simulink model "psbbridges"  (Simulink 6.0)
settings: Solver=FixedStepDiscrete  StartTime=0.0  StopTime=0.10  FixedStep=Ts  RelTol=1e-3  AbsTol=1e-3
PreLoadFcn:
  | assignin('base','Ts',[2e-6])
InitFcn:
  | powericon('psbinitsys',bdroot);
undefined symbols (not defined in the file or in its folder): D1, Delta, Ts
libraries: powerlib2 x16, powerlib_extras x5
settings Model: Creator=sybille  LastModifiedBy=batserve  ExtModeTrigMode=oneshot  ExtModeArmWhenConnect=off  ExtModeAutoUpdateStatusClock=off
settings DataIOCC: LimitDataPoints=off  SaveOutput=off  SaveTime=off  SignalLoggingName=sigsOut
settings OptimizationCC: BlockReduction=off  BooleanDataType=off
settings DebuggingCC: CheckExecutionContextPreStartOutputMsg=on  CheckExecutionContextRuntimeOutputMsg=on  SolverPrmCheckMsg=none
settings HardwareCC: TargetUnknown=on

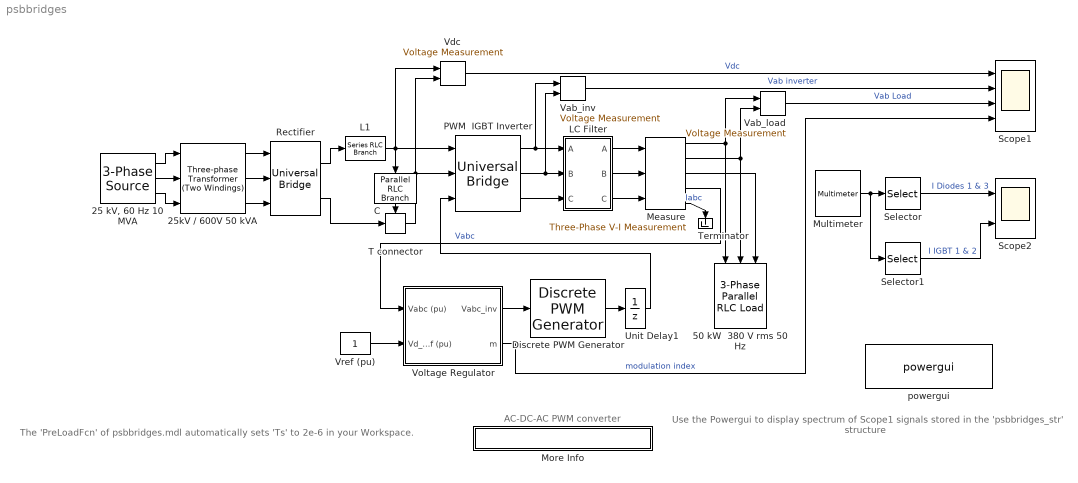
== system psbbridges ==
  note: AC-DC-AC PWM converter
  note: The 'PreLoadFcn' of psbbridges.mdl
      | automatically sets 'Ts' to 2e-6 in your Workspace.
  note: Use the Powergui to display
      | spectrum of Scope1 signals
      | stored in the  'psbbridges_str'
      | structure
  "25 kV, 60 Hz 10 MVA" : powerlib2/Electrical Sources/3-Phase Source  Tag=PoWeRsYsTeMbLoCk  V=25e3  Phi=0  F=60  InternalConnection=Yg  RLoff=on  R=25e3^2/10e6/5  L=25e3^2/10e6/377  Psc=10e6  Vbase=25e3  XRratio=5  PSBOutputType=111
  25kV / 600V 50 kVA : powerlib2/Elements/Three-phase Transformer (Two Windings)  Tag=PoWeRsYsTeMbLoCk  nominal=[ 50e3 , 60 ]  type1=Yg  params1=[ 25e3 , 0.004 , 0.02 ]  type2=Delta (D1)  params2=[ 600 , 0.004 , 0.02 ]  ynsat=off  rmag=200  lm=200  sat="[ 0,0  ;  0.005,1.2  ;  1.0,1.4 ]"  hyst=off  matfile='hysteresis'  sif=off  phi0=[ 0.8 , -0.8 , 0.7 ]  initialslopes=[+1 +1 +1]  mesure=None  PSBOutputType=1111
  50 kW  380 V rms 50 Hz : powerlib2/Elements/3-Phase Parallel RLC Load  Orientation=down  Vpp=380  fn=50  P3=50e3  QL3=0  QC3=0
  C : powerlib2/Elements/Parallel RLC Branch  Tag=PoWeRsYsTeMbLoCk  Orientation=down  a=inf  b=inf  c=5000e-06  mesure=None  PSBOutputType=1
  Discrete PWM Generator : powerlib_extras/Discrete  Control Blocks/Discrete PWM Generator  GeneratorMode="3-arm  bridge (6 pulses)"  Fc=2000  Ts=Ts  Internal=off  mIndex=0.4  Freq=60  Phase=0
  L1 : powerlib2/Elements/Series RLC Branch  Tag=PoWeRsYsTeMbLoCk  a=0  b=200e-6  c=inf  mesure=None  PSBOutputType=1
  LC Filter : Subsystem
  Measure : powerlib2/Measurements/Three-Phase V-I Measurement  Tag=PoWeRsYsTeMmEaSuReMeNt  VChoice=phase-to-ground  ualv=off  labelV=V1  Vpu=on  Vbase=380  IChoice=yes  ualc=off  labelC=I1  Ppu=off  Pbase=1e3  OutputType=Magnitude  PhasorSimulation=off  PSBequivalent=0  PSBOutputType=11100
  More Info : Subsystem
      mask Display: disp('? : Double click here for more info')
  Multimeter : powerlib2/Measurements/Multimeter  Tag=PoWeRsYsTeMmEaSuReMeNt  PhasorSimulation=off  OutputType=Magnitude  sel=[1 3 7 8]  L=12  Gain=[1 1 1 1]  yselected="{'Isw1: Rectifier','Isw3: Rectifier','Isw1: PWM  IGBT Inverter','Isw2: PWM  IGBT Inverter'};"  PSBOutputType=1  PSBequivalent=0  AxesSetting=[0,0.1,-100,100]  Display=0  SavedBlockNames=-11
  PWM  IGBT Inverter : powerlib2/Power Electronics/Universal Bridge  Tag=PoWeRsYsTeMbLoCk  arms=3  confi=ABC as output terminals  injcc=5000  cf=inf  device=IGBT / Diodes  Ron=1e-3  Lon=0  VFs="[  0.0  0.0  ]"  Vf=.8  gtoparameters=[ 1e-6 ,1e-6 ]  igbtparameters=[ 1e-6 , 2e-6 ]  mesure=Device currents  PSBOutputType=111
  Rectifier : powerlib2/Power Electronics/Universal Bridge  Tag=PoWeRsYsTeMbLoCk  arms=3  confi=ABC as input terminals  injcc=100  cf=0.1e-6  device=Diodes  Ron=1e-3  Lon=0  VFs="[  0.8  0.8  ]"  Vf=.8  gtoparameters=[ 10e-6 , 20e-6 ]  igbtparameters=[ 1e-6 , 2e-6 ]  mesure=Device currents  PSBOutputType=111
  Scope1 : Scope  NumInputPorts=4
      settings: TimeRange=0.1  YMin=0~-1500~-750~0.4  YMax=1100~1500~750~1.1  SaveName=psbbridges_str
  Scope2 : Scope  NumInputPorts=2
      settings: TimeRange=0.09999999999999999  YMin=-10~-125  YMax=100~125
  Selector : Selector  Elements=[1 2]  InputPortWidth=4
  Selector1 : Selector  Elements=[3 4]  InputPortWidth=4
  T connector : powerlib2/Connectors/T connector  Tag=PoWeRsYsTeMbLoCk  PSBOutputType=1
  Terminator : Terminator
      settings: Orientation=down
  Unit Delay1 : UnitDelay  SampleTime=Ts
  Vab_inv : powerlib2/Measurements/Voltage Measurement  Tag=PoWeRsYsTeMmEaSuReMeNt  PhasorSimulation=off  OutputType=Magnitude  PSBOutputType=0  PSBequivalent=0
  Vab_load : powerlib2/Measurements/Voltage Measurement  Tag=PoWeRsYsTeMmEaSuReMeNt  PhasorSimulation=off  OutputType=Magnitude  PSBOutputType=0  PSBequivalent=0
  Vdc : powerlib2/Measurements/Voltage Measurement  Tag=PoWeRsYsTeMmEaSuReMeNt  PhasorSimulation=off  OutputType=Magnitude  PSBOutputType=0  PSBequivalent=0
  Voltage Regulator : Subsystem  mask( Voltage Regulator){Kp=0.4, Ki=500, Ts=Ts}
      mask prompts: Kp "Proportional gain  Kp:"; Ki "Integral gain Ki:"; Ts "Sample time (s) :"
  "Vref (pu) " : Constant
  powergui : powerlib2/powergui  Frange=[0:2:500]  Ylog=off  Xlog=on  save=off  variable=ZData  structure=psbbridges_str  ZoomFFT=on  StartTime=0.1-2/50  cycles=2  DisplayStyle=off  fundamental=50  FreqAxis=off  MaxFrequency=7000  frequencyindice=1  frequencyindicesteady=1  RmsSteady=1  display=off  Ts=Ts  methode=off  frequency=60  echomessages=off
  wires:
  C/1 -> T connector/Enable
  T connector/1 -> PWM  IGBT Inverter/2, Vdc/2
  L1/1 -> PWM  IGBT Inverter/1, C/1, Vdc/1
  25kV / 600V 50 kVA/3 -> Rectifier/3
  "25 kV, 60 Hz 10 MVA"/1 -> 25kV / 600V 50 kVA/1
  "25 kV, 60 Hz 10 MVA"/2 -> 25kV / 600V 50 kVA/2
  "25 kV, 60 Hz 10 MVA"/3 -> 25kV / 600V 50 kVA/3
  25kV / 600V 50 kVA/2 -> Rectifier/2
  PWM  IGBT Inverter/1 -> Vab_inv/1, LC Filter/1(A)
  PWM  IGBT Inverter/2 -> Vab_inv/2, LC Filter/2(B)
  PWM  IGBT Inverter/3 -> LC Filter/3(C)
  LC Filter/1("A ") -> Measure/1
  LC Filter/2("B ") -> Measure/2
  LC Filter/3("C ") -> Measure/3
  Measure/3 -> 50 kW  380 V rms 50 Hz/3
  Measure/1 -> 50 kW  380 V rms 50 Hz/1, Vab_load/1
  Measure/2 -> 50 kW  380 V rms 50 Hz/2, Vab_load/2
  Measure/4 -> Voltage Regulator/1(Vabc (pu))  "Vabc"
  "Vref (pu) "/1 -> Voltage Regulator/2(Vd_ref (pu))
  Selector/1 -> Scope2/1  "I Diodes 1 & 3"
  Multimeter/1 -> Selector/1, Selector1/1
  Selector1/1 -> Scope2/2  "I IGBT 1 & 2"
  Measure/5 -> Terminator/1  "Iabc"
  25kV / 600V 50 kVA/1 -> Rectifier/1
  Rectifier/1 -> L1/1
  Rectifier/2 -> T connector/1
  Discrete PWM Generator/1 -> Unit Delay1/1
  Unit Delay1/1 -> PWM  IGBT Inverter/3
  Voltage Regulator/1(Vabc_inv) -> Discrete PWM Generator/1
  Voltage Regulator/2(m) -> Scope1/4  "modulation index"
  Vdc/1 -> Scope1/1  "Vdc"
  Vab_load/1 -> Scope1/3  "Vab Load"
  Vab_inv/1 -> Scope1/2  "Vab inverter"

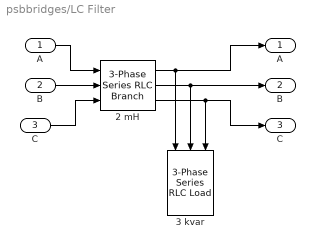
== system psbbridges/LC Filter ==
  A : Inport  Port=1  LatchInput=off
  B : Inport  Port=2  LatchInput=off
  C : Inport  Port=3  LatchInput=off
  "2 mH " : powerlib2/Elements/3-Phase Series RLC Branch   R=0  L=2e-3  C=inf
  3 kvar : powerlib2/Elements/3-Phase Series RLC Load  Orientation=down  Vpp=380  fn=50  P3=0  QL3=0  QC3=3e3
  "A " : Outport
  "B " : Outport  Port=2
  "C " : Outport  Port=3
  wires:
  B/1 -> "2 mH "/2
  A/1 -> "2 mH "/1
  C/1 -> "2 mH "/3
  "2 mH "/1 -> "A "/1, 3 kvar/1
  "2 mH "/2 -> "B "/1, 3 kvar/2
  "2 mH "/3 -> "C "/1, 3 kvar/3

== system psbbridges/More Info ==
  note: This example of AC-DC-AC converter illustrates use of Universal Bridge,
      |  Multimeter and Powergui  blocks as well as discrete control blocks of the Extras library
  note: Circuit Description
  note: Demonstration
  note: A  60 Hz, voltage source feeds a 50 Hz, 50 kW load through an  AC-DC-AC  converter.
      |
      | The 600V, 60 Hz voltage obtained at secondary of the Wye/Delta transformer is first rectified by a six pulse diode bridge.
      | The filtered DC voltage is applied to an IGBT two-level inverter generating 50 Hz.
      | The IGBT inverter uses Pulse Width Modulation (PWM) at a 2 kHz carrier frequency.
      | The circuit is discretized at a sample time of 2 us
      |
      | The load voltage is regulated  at 1 pu (380 V rms) by a PI voltage regulator using abc_to_dq and dq_to_abc transfomations.
      | The first output of the voltage regulator is a vector containing the three modulating signals used by the PMW Generator
      | to generate the 6 IGBT pulses. The second output returns the modulation index.
      |
      | The Discrete 3-Phase PWM Pulse Generator  is available in the Extras/Discrete Control Blocks library.
      | The voltage regulator has been  built from blocks of the Extras/Measurements and Extras/ Discrete Control libraries
      |
      | The Multimeter block is used to observe diode and IGBT currents.
      | In order to allow further signal processing, signals displayed on  Scope1  block  (sampled at simulation sampling rate of 2us )
      | are stored in a  variable named 'psbbridges_str' (structure with time) .
  note: Start the simulation. After a transient period of approximately  50 ms, the system reaches a steady state.
      | Observe  voltage waveforms at  DC bus, inverter output  and load on Scope1.
      | The harmonics generated by the inverter around around multiples of 2 kHz are filtered by the  LC filter.
      |
      | As expected the peak value of the load voltage is 537 V (380 Vrms).
      | In steady state the mean value of the  modulation index is m = 0.80 and the mean value of the  DC  voltage is 778 V.
      | The fundamental component of 50 Hz voltage burried in the chopped inverter voltage is therefore:
      | Vab = 778 V * 0.612 * 0.80 = 381 V rms
      |
      | Once  simulation is completed, open the Powergui and select  'FFT Analysis' to display the 0 - 7000 Hz frequency spectrum of signals saved
      | in the 'psbbridges_str' structure. The FFT will be performed on  a 2-cycle window starting at t=0.1-2/50 (last 2 cycles of recording).
      | Select input labeled 'Vab Load' . Click on Display and observe the frequency spectrum of last 2 cycles.
      | Notice harmonics around multiples of the 2 kHz carrier frequency. Maximum harmonic is 1.4 % of fundamental and THD is 2%.
      |
      | Observe diode currents on trace 1 of Scope2, showing commutation from  diode 1 to diode 3.  Also observe on trace 2 currents in
      | switches 1 and 2 of the IGBT/Diode bridge (upper and lower switches connected to phase A). These two currents are complementary.
      | A positive current indicates a current flowing in the IGBT, whereas a negative current indicates a current flowing in the antiparallel diode.
  note: G. Sybille (Hydro-Quebec)

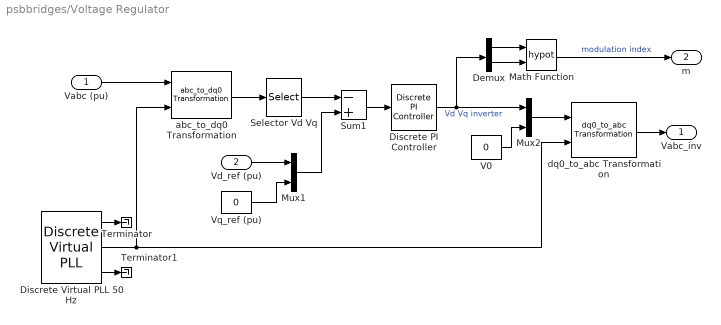
== system psbbridges/Voltage Regulator ==
  Vabc (pu) : Inport  Port=1  LatchInput=off
  Vd_ref (pu) : Inport  Port=2  LatchInput=off
  Demux : Demux  Outputs=2
  Discrete PI Controller : powerlib_extras/Discrete  Control Blocks/Discrete PI Controller  Kp=Kp  Ki=Ki  Par_Limits=[1 -1]  Init=0  Ts=Ts
  Discrete Virtual PLL 50 Hz : powerlib_extras/Discrete  Control Blocks/Discrete Virtual PLL  Freq=50  Phase=0  Ts=Ts
  Math Function : Math  Operator=hypot  SaturateOnIntegerOverflow=on
  Mux1 : Mux  Inputs=2
  Mux2 : Mux  Inputs=2
  Selector Vd Vq : Selector  Elements=[1 2]  InputPortWidth=3
  Sum1 : Sum  Inputs=-+  SaturateOnIntegerOverflow=on  InputSameDT=on
  Terminator : Terminator
  Terminator1 : Terminator
  V0 : Constant  Value=0
  Vq_ref (pu) : Constant  Value=0
  abc_to_dq0 Transformation : powerlib_extras/Measurements/abc_to_dq0 Transformation
  dq0_to_abc Transformation : powerlib_extras/Measurements/dq0_to_abc Transformation
  Vabc_inv : Outport
  m : Outport  Port=2
  wires:
  abc_to_dq0 Transformation/1 -> Selector Vd Vq/1
  Vabc (pu)/1 -> abc_to_dq0 Transformation/1
  Selector Vd Vq/1 -> Sum1/1
  Sum1/1 -> Discrete PI Controller/1
  Mux2/1 -> dq0_to_abc Transformation/1
  V0/1 -> Mux2/2
  dq0_to_abc Transformation/1 -> Vabc_inv/1
  Discrete Virtual PLL 50 Hz/2 -> abc_to_dq0 Transformation/2, dq0_to_abc Transformation/2
  Vd_ref (pu)/1 -> Mux1/1
  Vq_ref (pu)/1 -> Mux1/2
  Mux1/1 -> Sum1/2
  Discrete Virtual PLL 50 Hz/1 -> Terminator/1
  Discrete Virtual PLL 50 Hz/3 -> Terminator1/1
  Discrete PI Controller/1 -> Demux/1, Mux2/1  "Vd Vq inverter"
  Demux/1 -> Math Function/1
  Demux/2 -> Math Function/2
  Math Function/1 -> m/1  "modulation index"
